simulink model "VehControl"  (R2021a)
settings: Solver=ode1  StartTime=0.0  StopTime=inf  FixedStep=0.001  RelTol=1e-3
PreLoadFcn:
  | vehicle = 'Car'; if ~length(which('cmself')), cmenv; end
  | VehControl_bus
InitFcn:
  | vehicle = 'Car'; if ~length(which('cmself')), cmenv; end
  | VehControl_bus
Description:
  | CarMaker Plug-in Model Target
settings Model: Creator=giri  LastModifiedBy=giri
settings RTWCC: Description=CarMaker Plug-in Model Target  SystemTargetFile=CarMaker.tlc  TemplateMakefile=CarMaker_unix-linux64.tmf
settings CodeAppCC: MaxIdLength=127
settings STFCustomTargetCC: TargetLangStandard=C99 (ISO)  CombineOutputUpdateFcns=on  MatFileLogging=on  CodeInterfacePackaging=Reusable function  GRTInterface=off  GenerateAllocFcn=on  UseToolchainInfoCompliant=off  SystemTargetFile=CarMaker.tlc
settings GRTTargetCC: ParMdlRefBuildCompliant=off  CompOptLevelCompliant=off  ConcurrentExecutionCompliant=off  CodeInterfacePackaging=Reusable function  CPPClassGenCompliant=off  GenerateAllocFcn=on  UseToolchainInfoCompliant=off

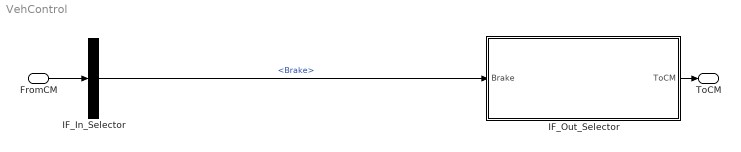
== system VehControl ==
  FromCM : Inport  OutDataTypeStr=Bus: cmVehicleControlIn
  IF_In_Selector : BusSelector  OutputSignals=Brake
  IF_Out_Selector : Subsystem  mask(Signal Selection){}
      mask help: Signal Selection Block
      settings: OpenFcn=cmSignalSelect('SignalSelection_CB',gcb)
  ToCM : Outport  OutDataTypeStr=Bus: cmVehicleControlOut
  wires:
  FromCM/1 -> IF_In_Selector/1
  IF_In_Selector/1 -> IF_Out_Selector/1(Brake)  "<Brake>"
  IF_Out_Selector/1(ToCM) -> ToCM/1

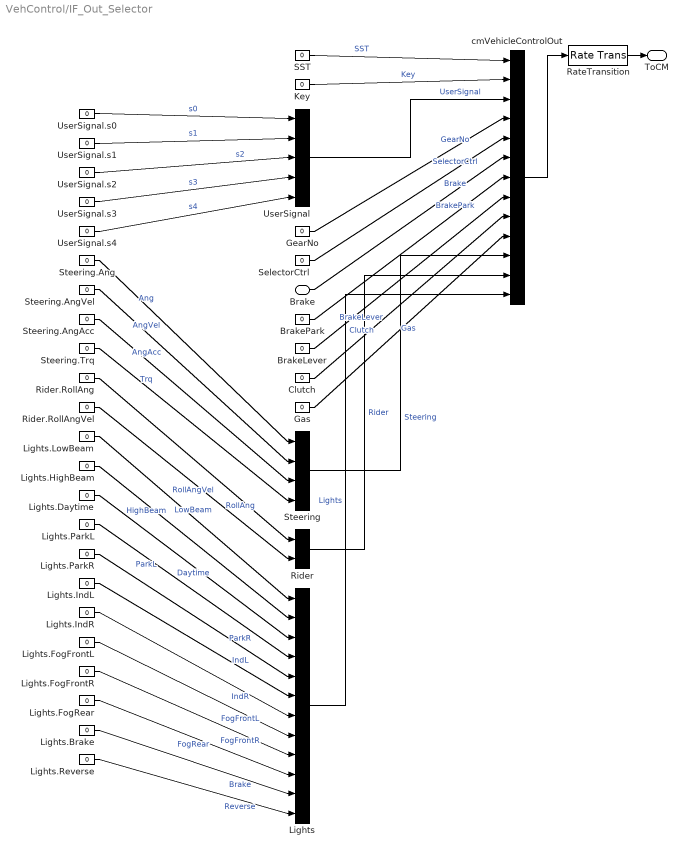
== system VehControl/IF_Out_Selector ==
  Brake : Inport
  BrakeLever : Constant  Value=0
  BrakePark : Constant  Value=0
  Clutch : Constant  Value=0
  Gas : Constant  Value=0
  GearNo : Constant  Value=0
  Key : Constant  Value=0
  Lights : BusCreator  Inputs=12
  Lights.Brake : Constant  Value=0
  Lights.Daytime : Constant  Value=0
  Lights.FogFrontL : Constant  Value=0
  Lights.FogFrontR : Constant  Value=0
  Lights.FogRear : Constant  Value=0
  Lights.HighBeam : Constant  Value=0
  Lights.IndL : Constant  Value=0
  Lights.IndR : Constant  Value=0
  Lights.LowBeam : Constant  Value=0
  Lights.ParkL : Constant  Value=0
  Lights.ParkR : Constant  Value=0
  Lights.Reverse : Constant  Value=0
  RateTransition : RateTransition  OutPortSampleTime=str2num(get_param(bdroot,'FixedStep'))
  Rider : BusCreator  Inputs=2
  Rider.RollAng : Constant  Value=0
  Rider.RollAngVel : Constant  Value=0
  SST : Constant  Value=0
  SelectorCtrl : Constant  Value=0
  Steering : BusCreator  Inputs=4
  Steering.Ang : Constant  Value=0
  Steering.AngAcc : Constant  Value=0
  Steering.AngVel : Constant  Value=0
  Steering.Trq : Constant  Value=0
  UserSignal : BusCreator  Inputs=5
  UserSignal.s{0..4} (5 alike) : Constant  Value=0
  cmVehicleControlOut : BusCreator  Inputs=13
  ToCM : Outport
  wires:
  RateTransition/1 -> ToCM/1
  cmVehicleControlOut/1 -> RateTransition/1
  SST/1 -> cmVehicleControlOut/1  "SST"
  Key/1 -> cmVehicleControlOut/2  "Key"
  UserSignal/1 -> cmVehicleControlOut/3  "UserSignal"
  UserSignal.s0/1 -> UserSignal/1  "s0"
  UserSignal.s1/1 -> UserSignal/2  "s1"
  UserSignal.s2/1 -> UserSignal/3  "s2"
  UserSignal.s3/1 -> UserSignal/4  "s3"
  UserSignal.s4/1 -> UserSignal/5  "s4"
  GearNo/1 -> cmVehicleControlOut/4  "GearNo"
  SelectorCtrl/1 -> cmVehicleControlOut/5  "SelectorCtrl"
  BrakePark/1 -> cmVehicleControlOut/7  "BrakePark"
  BrakeLever/1 -> cmVehicleControlOut/8  "BrakeLever"
  Clutch/1 -> cmVehicleControlOut/9  "Clutch"
  Gas/1 -> cmVehicleControlOut/10  "Gas"
  Steering/1 -> cmVehicleControlOut/11  "Steering"
  Steering.Ang/1 -> Steering/1  "Ang"
  Steering.AngVel/1 -> Steering/2  "AngVel"
  Steering.AngAcc/1 -> Steering/3  "AngAcc"
  Steering.Trq/1 -> Steering/4  "Trq"
  Rider/1 -> cmVehicleControlOut/12  "Rider"
  Rider.RollAng/1 -> Rider/1  "RollAng"
  Rider.RollAngVel/1 -> Rider/2  "RollAngVel"
  Lights/1 -> cmVehicleControlOut/13  "Lights"
  Lights.LowBeam/1 -> Lights/1  "LowBeam"
  Lights.HighBeam/1 -> Lights/2  "HighBeam"
  Lights.Daytime/1 -> Lights/3  "Daytime"
  Lights.ParkL/1 -> Lights/4  "ParkL"
  Lights.ParkR/1 -> Lights/5  "ParkR"
  Lights.IndL/1 -> Lights/6  "IndL"
  Lights.IndR/1 -> Lights/7  "IndR"
  Lights.FogFrontL/1 -> Lights/8  "FogFrontL"
  Lights.FogFrontR/1 -> Lights/9  "FogFrontR"
  Lights.FogRear/1 -> Lights/10  "FogRear"
  Lights.Brake/1 -> Lights/11  "Brake"
  Lights.Reverse/1 -> Lights/12  "Reverse"
  Brake/1 -> cmVehicleControlOut/6  "Brake"
